simulink model "inverse_kinematics"  (R2019a)
settings: Solver=FixedStepAuto  StartTime=0.0  StopTime=10.0  FixedStep=0.01  RelTol=1e-3
model workspace: external: MATLAB File D:\RIC_LAB\SolidWork_Ric\Simulink\robot_DataFile1.m (data not in the file)
undefined symbols (not defined in the file): smiData, X, Y, Z
libraries: sm_lib x40, nesl_utility x14, simulink_extras x12, simulink x1
(part 2 of 2)

== matlab function inverse_kinematics/TAM GIÁC ==
  data: x output; t input; y output; P input; T input; V input; cycle input
function [x, y] = trajectory(t,P,T,V,cycle)
    cycle_time = cycle * T(end);
    t_mod = mod(t, T(end));
    x = P(1,1);
    y = P(1,2);
    if t_mod < T(1)
        return;
    elseif t >= cycle_time
        x = P(end,1);
        y = P(end,2);
        return;
    end

    for i = 1:length(T)-1
        if t_mod >= T(i) && t_mod <= T(i+1)
            P0 = P(i,:);   Pf = P(i+1,:);
            v0 = V(i,:);   vf = V(i+1,:);
            t0 = T(i);     tf = T(i+1);
            
            a0 = P0;
            a1 = v0;
            a2 = (3/(tf-t0)^2) * (Pf - P0) - (2/(tf-t0)) * v0 - (1/(tf-t0)) * vf;
            a3 = (-2/(tf-t0)^3) * (Pf - P0) + (1/(tf-t0)^2) * (vf + v0);
            
            % Tính vị trí
            dt = t_mod - t0;
            x = a0(1) + a1(1)*dt + a2(1)*dt^2 + a3(1)*dt^3;
            y = a0(2) + a1(2)*dt + a2(2)*dt^2 + a3(2)*dt^3;
            return;
        end
    end
end

== matlab function inverse_kinematics/FK ==
  data: q1 input; x output; q2 input; q3 input; y output; z output
%% Programmed by Nguyen Ngoc Gia Huy
function [x,y,z] = FK(q1,q2,q3)
    % Thông số
    L1 = 16; L2 = 7; L3 = 15; L4 = 15;
    % [x;y;z]
    x = cos(q1)*(L2 + L3*cos(q2) + L4*cos(q2 + q3));
    y = sin(q1)*(L2 + L3*cos(q2) + L4*cos(q2 + q3));
    z = L1 + L3*sin(q2) + L4*sin(q2 + q3);
end

== matlab function inverse_kinematics/IK ==
  data: x input; q1 output; y input; z input; solution input; q2 output; q3 output
function [q1,q2,q3] = IK(x, y, z, solution)
    % Khai báo chiều dài các liên kết
    l1 = 16; l2 = 7; l3 = 15; l4 = 15;
    q1 = NaN; q2 = NaN; q3 = NaN;

    %% Tính q1
    q11 = atan2(y, x);

    %% Tính q3
    A = sqrt(x^2 + y^2) - l2;
    B = z - l1;
    D = (A^2 + B^2 - l3^2 - l4^2) / (2 * l3 * l4);
    % Kiểm tra điều kiện tồn tại
    if abs(D) > 1
        return;  % Không có nghiệm thực
    end

    q31 = atan2(sqrt(1 - D^2), D);
    q32 = atan2(-sqrt(1 - D^2), D);

    %% Tính q2
    E1 = l3 + l4 * cos(q31); F1 = l4 * sin(q31);
    E2 = l3 + l4 * cos(q32); F2 = l4 * sin(q32);

    q21 = atan2(B * E1 - A * F1, A * E1 + B * F1);
    q22 = atan2(B * E2 - A * F2, A * E2 + B * F2);

    %% 2 bộ nghiệm
    if solution==1
        q1 = q11;
        q2 = q21;
        q3 = q31;
    elseif solution==2
        q1 = q11;
        q2 = q22;
        q3 = q32;
    else
    end

end

== matlab function inverse_kinematics/ĐƯỜNG THẲNG ==
  data: x output; t input; y output; P0 input; v0 input; t0 input; Pf input; vf input; tf input; cycle input
function [x, y] = TrajectoryPlanning(t, P0, v0, t0, Pf, vf, tf, cycle)
    duration = tf - t0;              % Thời gian của 1 chu kỳ
    total_time = cycle * duration;  % Tổng thời gian cần chạy

    if t < t0
        x = P0(1);
        y = P0(2);
        return;

    elseif t >= t0 + total_time
        x = Pf(1);
        y = Pf(2);
        return;

    else
        % Tính thời gian tương đối trong 1 chu kỳ
        t_relative = mod(t - t0, duration);

        % Hệ số quỹ đạo (bậc 3)
        a10 = P0(1);
        a20 = P0(2);
        a11 = v0(1);
        a21 = v0(2);
        a12 = 3 / duration^2 * (Pf(1) - P0(1)) - 2 / duration * v0(1) - 1 / duration * vf(1);
        a22 = 3 / duration^2 * (Pf(2) - P0(2)) - 2 / duration * v0(2) - 1 / duration * vf(2);
        a13 = -2 / duration^3 * (Pf(1) - P0(1)) + 1 / duration^2 * (vf(1) + v0(1));
        a23 = -2 / duration^3 * (Pf(2) - P0(2)) + 1 / duration^2 * (vf(2) + v0(2));

        % Tính vị trí tại thời điểm tương đối trong chu kỳ
        x = a10 + a11 * t_relative + a12 * t_relative^2 + a13 * t_relative^3;
        y = a20 + a21 * t_relative + a22 * t_relative^2 + a23 * t_relative^3;
    end
end
